simulink library "csu_kfo_kalman_filter_output_mtv_lib"  (R2014b)
settings: Solver=ode45  StartTime=0.0  StopTime=10.0  RelTol=1e-3
libraries: util_common_lib x7, util_quat_lib x2, util_info_lib x1
settings Model: Creator=escrane  LastModifiedBy=tgorton

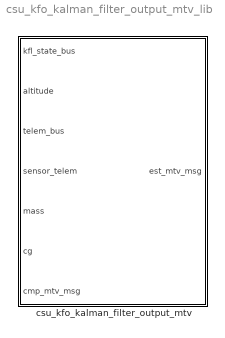
== system csu_kfo_kalman_filter_output_mtv_lib ==
  csu_kfo_kalman_filter_output_mtv : Subsystem

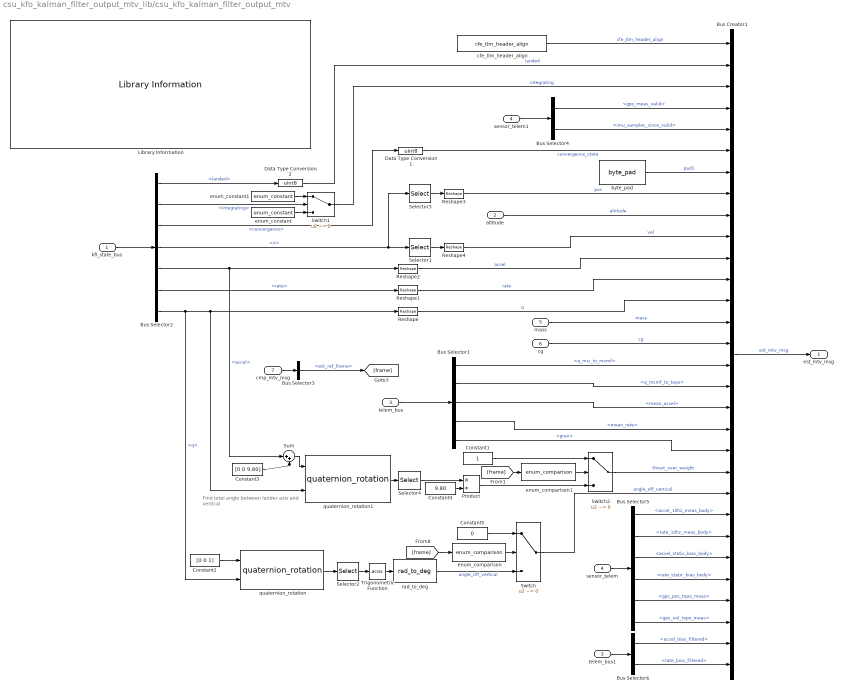
== system csu_kfo_kalman_filter_output_mtv_lib/csu_kfo_kalman_filter_output_mtv ==
  note: Find total angle between lander
      | axis and vertical
  kfl_state_bus : Inport
  altitude : Inport  Port=2
  telem_bus : Inport  Port=3
  sensor_telem : Inport  Port=4
  mass : Inport  Port=5
  cg : Inport  Port=6
  cmp_mtv_msg : Inport  Port=7
  Bus Creator1 : BusCreator  Inputs=30  OutDataTypeStr=Bus: est_mtv_msg  NonVirtualBus=on
  Bus Selector1 : BusSelector  OutputSignals=q_mci_to_mcmf,q_mcmf_to_topo,mean_accel,mean_rate,grav
  Bus Selector2 : BusSelector  OutputSignals=landed,integrating,convergence,x,accel,rate,q
  Bus Selector3 : BusSelector  OutputSignals=est_ref_frame
  Bus Selector4 : BusSelector  OutputSignals=gps_telem.gps_meas_valid,imu_telem.imu_samples_since_valid
  Bus Selector5 : BusSelector  OutputSignals=imu_telem.accel_10hz_meas_body,imu_telem.rate_10hz_meas_body,imu_telem.accel_static_bias_body,imu_telem.rate_static_bias_body,gps_telem.gps_pos_topo_meas,gps_telem.gps_vel_topo_meas
  Bus Selector6 : BusSelector  OutputSignals=accel_bias_filtered,rate_bias_filtered
  Constant1 : Constant  OutDataTypeStr=double
  Constant2 : Constant  Value=[0 0 1]  OutDataTypeStr=double
  Constant3 : Constant  Value=[0 0 9.80]  OutDataTypeStr=double
  Constant4 : Constant  Value=9.80  OutDataTypeStr=double
  Constant5 : Constant  Value=0  OutDataTypeStr=double
  Data Type Conversion1 : DataTypeConversion  OutDataTypeStr=uint8
  Data Type Conversion2 : DataTypeConversion  OutDataTypeStr=uint8
  Library Information : util_info_lib/Library Information  owner='escrane'
  Product : Product  Inputs=*/
  Reshape{,1..4} (5 alike) : Reshape
  Selector1 : Selector  InputPortWidth=kfl_n_state  Indices=kfl_vel_index
  Selector2 : Selector  InputPortWidth=3  Indices=3
  Selector3 : Selector  InputPortWidth=kfl_n_state  Indices=kfl_pos_index
  Selector4 : Selector  InputPortWidth=3  Indices=3
  Sum : Sum  Inputs=|++
  Switch : Switch  Criteria=u2 ~= 0
  Switch1 : Switch  Criteria=u2 ~= 0
  Switch2 : Switch  Criteria=u2 ~= 0
  Trigonometric Function : Trigonometry  Operator=acos
  byte_pad : util_common_lib/byte_pad  n_bytes=7
  cfe_tlm_header_align : util_common_lib/cfe_tlm_header_align
  enum_comparison : util_common_lib/enum_comparison  comparison_type=~=
  enum_comparison1 : util_common_lib/enum_comparison  comparison_type=~=
  enum_constant : util_common_lib/enum_constant
  enum_constant1 : util_common_lib/enum_constant
  quaternion_rotation : util_quat_lib/quaternion_rotation  SystemSampleTime=-1
  quaternion_rotation1 : util_quat_lib/quaternion_rotation  SystemSampleTime=-1
  rad_to_deg : util_common_lib/rad_to_deg  SystemSampleTime=-1
  sensor_telem1 : InportShadow  Port=4
  telem_bus1 : InportShadow  Port=3
  est_mtv_msg : Outport
  wires:
  Bus Selector1/5 -> Bus Creator1/20  "<grav>"
  Bus Selector5/6 -> Bus Creator1/28  "<gps_vel_topo_meas>"
  Bus Selector6/2 -> Bus Creator1/30  "<rate_bias_filtered>"
  Bus Selector6/1 -> Bus Creator1/29  "<accel_bias_filtered>"
  telem_bus1/1 -> Bus Selector6/1
  [frame] -> enum_comparison1/1
  [frame] -> enum_comparison/1
  Bus Selector3/1 -> [frame]  "<est_ref_frame>"
  Constant1/1 -> Switch2/1
  Product/1 -> Switch2/3
  enum_comparison1/1 -> Switch2/2
  enum_constant1/1 -> Switch1/1
  enum_constant/1 -> Switch1/3
  Bus Selector5/4 -> Bus Creator1/26  "<rate_static_bias_body>"
  Bus Selector5/3 -> Bus Creator1/25  "<accel_static_bias_body>"
  byte_pad/1 -> Bus Creator1/7  "pad1"
  Switch1/1 -> Bus Creator1/3  "integrating"
  Bus Selector2/2 -> Switch1/2  "<integrating>"
  Bus Selector5/5 -> Bus Creator1/27  "<gps_pos_topo_meas>"
  Bus Selector5/2 -> Bus Creator1/24  "<rate_10hz_meas_body>"
  Bus Selector5/1 -> Bus Creator1/23  "<accel_10hz_meas_body>"
  Bus Selector4/2 -> Bus Creator1/5  "<imu_samples_since_valid>"
  Bus Selector4/1 -> Bus Creator1/4  "<gps_meas_valid>"
  sensor_telem1/1 -> Bus Selector4/1
  sensor_telem/1 -> Bus Selector5/1
  Data Type Conversion1/1 -> Bus Creator1/6  "convergence_state"
  Bus Selector2/3 -> Data Type Conversion1/1  "<convergence>"
  cmp_mtv_msg/1 -> Bus Selector3/1
  Constant5/1 -> Switch/1
  rad_to_deg/1 -> Switch/3  "angle_off_vertical"
  enum_comparison/1 -> Switch/2
  Switch/1 -> Bus Creator1/22  "angle_off_vertical"
  Switch2/1 -> Bus Creator1/21  "thrust_over_weight"
  Constant4/1 -> Product/2
  Selector4/1 -> Product/1
  quaternion_rotation1/1 -> Selector4/1
  Constant3/1 -> Sum/2
  Sum/1 -> quaternion_rotation1/1
  Trigonometric Function/1 -> rad_to_deg/1
  Selector2/1 -> Trigonometric Function/1
  quaternion_rotation/1 -> Selector2/1
  Constant2/1 -> quaternion_rotation/1
  Bus Selector1/4 -> Bus Creator1/19  "<mean_rate>"
  Bus Selector1/3 -> Bus Creator1/18  "<mean_accel>"
  Bus Selector1/1 -> Bus Creator1/16  "<q_mci_to_mcmf>"
  Bus Selector1/2 -> Bus Creator1/17  "<q_mcmf_to_topo>"
  telem_bus/1 -> Bus Selector1/1
  cg/1 -> Bus Creator1/15  "cg"
  mass/1 -> Bus Creator1/14  "mass"
  kfl_state_bus/1 -> Bus Selector2/1
  cfe_tlm_header_align/1 -> Bus Creator1/1  "cfe_tlm_header_align"
  Bus Selector2/1 -> Data Type Conversion2/1  "<landed>"
  Reshape2/1 -> Bus Creator1/11  "accel"
  Bus Creator1/1 -> est_mtv_msg/1  "est_mtv_msg"
  Bus Selector2/7 -> Reshape/1, quaternion_rotation1/2, quaternion_rotation/2  "<q>"
  Bus Selector2/6 -> Reshape1/1  "<rate>"
  Bus Selector2/5 -> Reshape2/1, Sum/1  "<accel>"
  Selector1/1 -> Reshape4/1
  Bus Selector2/4 -> Selector1/1, Selector3/1  "<x>"
  Reshape/1 -> Bus Creator1/13  "q"
  Reshape1/1 -> Bus Creator1/12  "rate"
  Reshape4/1 -> Bus Creator1/10  "vel"
  Reshape3/1 -> Bus Creator1/8  "pos"
  Selector3/1 -> Reshape3/1
  Data Type Conversion2/1 -> Bus Creator1/2  "landed"
  altitude/1 -> Bus Creator1/9  "altitude"
